simulink model "doc_agc_received_signal_amplitude"  (R2014a)
settings: Solver=FixedStepDiscrete  StartTime=0.0  StopTime=2e3  RelTol=1e-3
libraries: commrfcorlib x1, commdigbbndpm3 x1, commrandsrc2 x1
settings Model: Creator=The MathWorks Inc.
settings DebuggingCC: UnderspecifiedInitializationDetection=Classic  StateNameClashWarn=warning

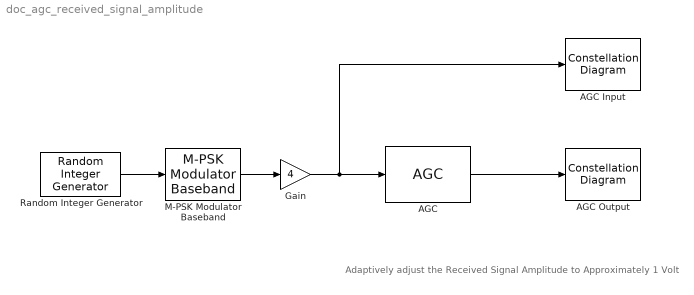
== system doc_agc_received_signal_amplitude ==
  note: Adaptively adjust the Received Signal Amplitude to Approximately 1 Volt
  AGC : commrfcorlib/AGC  SimulateUsing=Code generation  DetectorMethod=Rectifier  LoopMethod=Linear  UpdatePeriod=100  StepSize=0.1  MaximumGain=30  GainOutputPort=off
  AGC Input : ConstellationDiagram  Tag=ScatterPlot
  AGC Output : ConstellationDiagram  Tag=ScatterPlot
  Gain : Gain  Gain=4
  M-PSK Modulator Baseband : commdigbbndpm3/M-PSK Modulator Baseband  M=4  InType=Integer  Enc=Gray  Mapping=[0:7]  Ph=pi/4  outDtype=double  outWordLen=16  outUDDataType=sfix(16)  outFracLenMode=Best precision  outFracLen=15
  Random Integer Generator : commrandsrc2/Random Integer Generator  mul=4  seed=37  Ts=1  frameBased=on  sampPerFrame=1000  orient=off  outDataType=double
  wires:
  Random Integer Generator/1 -> M-PSK Modulator Baseband/1
  M-PSK Modulator Baseband/1 -> Gain/1
  AGC/1 -> AGC Output/1
  Gain/1 -> AGC Input/1, AGC/1
